simulink library "Lib_Local"  (R2023a)
settings: Solver=VariableStepAuto  StartTime=0.0  StopTime=10.0  RelTol=1e-3
settings Model: Creator=62555  LastModifiedBy=62555

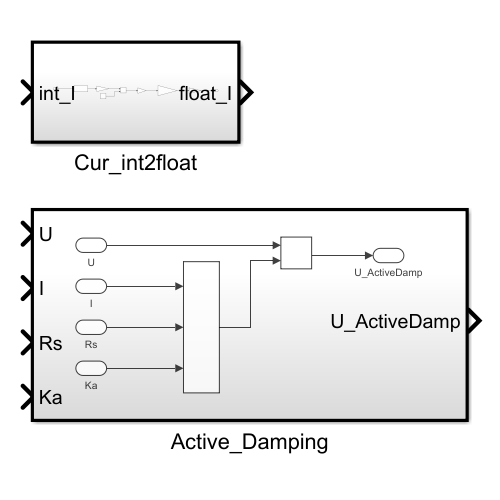
[thumbnail: Simulink's stored preview of the top-level diagram]
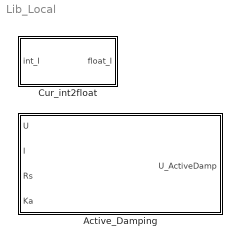
== system Lib_Local ==
  Active_Damping : Subsystem  TreatAsAtomicUnit=on  RTWFileName=Lib_Local
      settings: RTWFcnNameOpts=Use subsystem name  RTWFileNameOpts=User specified
  Cur_int2float : Subsystem  TreatAsAtomicUnit=on  RTWFileName=Lib_Local
      settings: RTWFcnNameOpts=Use subsystem name  RTWFileNameOpts=User specified

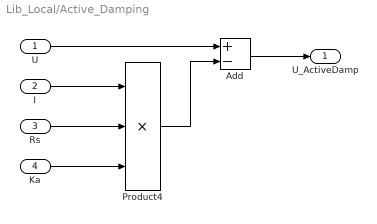
== system Lib_Local/Active_Damping ==
  U : Inport
  I : Inport  Port=2
  Rs : Inport  Port=3
  Ka : Inport  Port=4
  Add : Sum  Inputs=+-
  Product4 : Product  Inputs=3
  U_ActiveDamp : Outport
  wires:
  Product4/1 -> Add/2
  Rs/1 -> Product4/2
  U/1 -> Add/1
  Add/1 -> U_ActiveDamp/1
  I/1 -> Product4/1
  Ka/1 -> Product4/3

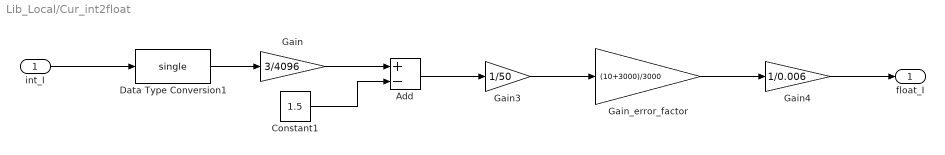
== system Lib_Local/Cur_int2float ==
  int_I : Inport
  Add : Sum  Inputs=+-
  Constant1 : Constant  Value=1.5  OutDataTypeStr=single  SampleTime=-1
  Data Type Conversion1 : DataTypeConversion  OutDataTypeStr=single  SaturateOnIntegerOverflow=off  RndMeth=Floor
  Gain : Gain  Gain=3/4096
  Gain3 : Gain  Gain=1/50
  Gain4 : Gain  Gain=1/0.006
  Gain_error_factor : Gain  Gain=(10+3000)/3000
  float_I : Outport
  wires:
  Add/1 -> Gain3/1
  Gain4/1 -> float_I/1
  Constant1/1 -> Add/2
  Gain/1 -> Add/1
  int_I/1 -> Data Type Conversion1/1
  Data Type Conversion1/1 -> Gain/1
  Gain3/1 -> Gain_error_factor/1
  Gain_error_factor/1 -> Gain4/1
